simulink model "p_damp_model_p_human"  (R2020b)
settings: Solver=VariableStepAuto  StartTime=0.0  StopTime=200  RelTol=1e-3
values from neighbouring files (symbols this model uses):
  A = [[0 1], ... (first row only)    [p_damp.m]
  A1 = [[0 1], ... (first row only)    [p_damp.m]
  B = [0, ... (first row only)    [p_damp.m]
  B1 = [0, ... (first row only)    [p_damp.m]
  Bl = sqrt(b)*alpha    [p_damp.m]
  Br = Bl*1    [p_damp.m]
  C = [[1 0], ... (first row only)    [p_damp.m]
  C1 = [[1 0], ... (first row only)    [p_damp.m]
  D = [0, ... (first row only)    [p_damp.m]
  D1 = [0, ... (first row only)    [p_damp.m]
  Kl = 0.4    [p_damp.m]
  Kr = 1.1*Kl    (= 0.44)    [p_damp.m]
  stp = 10    [p_damp.m]
  stp_end = 25    [p_damp.m]
  stp_start = 5    [p_damp.m]
  Tl = 2.5    [p_damp.m]
  torque_ratio = 5/8    (= 0.625)    [p_damp.m]
  Tr = 2.5    [p_damp.m]
settings Model: Creator=tammer  LastModifiedBy=tammer

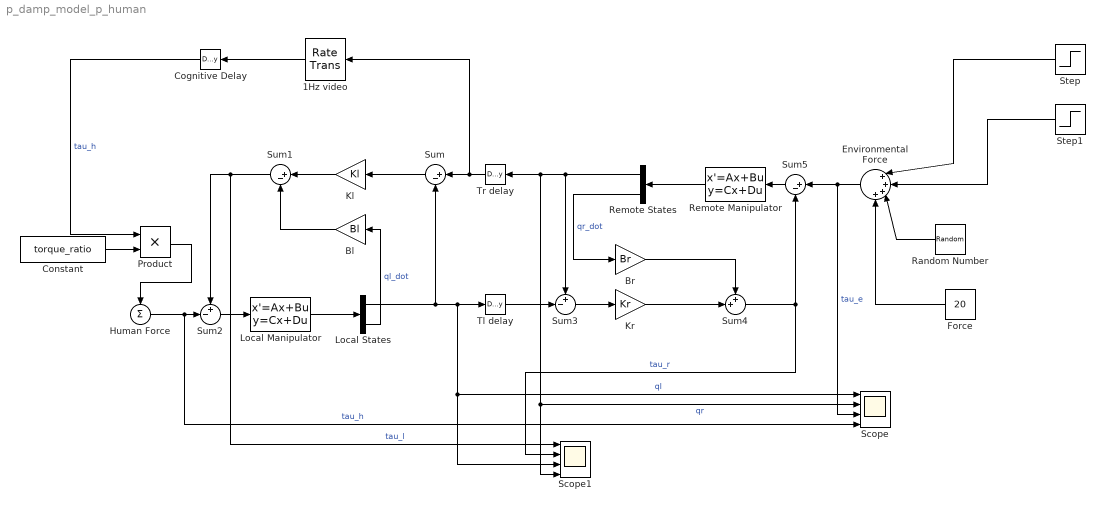
== system p_damp_model_p_human ==
  1Hz video : RateTransition  OutPortSampleTime=1
  Bl : Gain  Gain=Bl
  Br : Gain  Gain=Br
  Cognitive Delay : TransportDelay  DelayTime=.5
  Constant : Constant  Value=torque_ratio
  Environmental Force : Sum  Inputs=|++++
  Force : Constant  Value=20
  Human Force : Sum  Inputs=+|
  Kl : Gain  Gain=Kl
  Kr : Gain  Gain=Kr
  Local Manipulator : StateSpace  A=A  B=B  C=C  D=D  InitialCondition=0
  Local States : Demux  Outputs=2
  Product : Product
  Random Number : RandomNumber  Variance=2  Seed=6  SampleTime=0.1
  Remote Manipulator : StateSpace  A=A1  B=B1  C=C1  D=D1  InitialCondition=0
  Remote States : Demux  Outputs=2
  Scope : Scope  NumInputPorts=4
  Scope1 : Scope  NumInputPorts=4
  Step : Step  Time=stp_start  After=stp  SampleTime=0
  Step1 : Step  Time=stp_end  After=-stp  SampleTime=0
  Sum : Sum  Inputs=|+-
  Sum1 : Sum  Inputs=|+-
  Sum2 : Sum  Inputs=+-|
  Sum3 : Sum  Inputs=+-|
  Sum4 : Sum  Inputs=++|
  Sum5 : Sum  Inputs=|+-
  Tl delay : TransportDelay  DelayTime=Tl
  Tr delay : TransportDelay  DelayTime=Tr
  wires:
  Kl/1 -> Sum1/1
  Sum/1 -> Kl/1
  Sum3/1 -> Kr/1
  Environmental Force/1 -> Scope/3, Sum5/1  "tau_e"
  Tl delay/1 -> Sum3/2
  Sum2/1 -> Local Manipulator/1
  Sum5/1 -> Remote Manipulator/1
  Remote Manipulator/1 -> Remote States/1
  Remote States/1 -> Scope1/4, Scope/2, Tr delay/1, Sum3/1  "qr"
  Local Manipulator/1 -> Local States/1
  Local States/1 -> Tl delay/1, Scope1/3, Scope/1, Sum/2  "ql"
  Bl/1 -> Sum1/2
  Sum1/1 -> Sum2/1, Scope1/1  "tau_l"
  Kr/1 -> Sum4/2
  Br/1 -> Sum4/1
  Sum4/1 -> Sum5/2, Scope1/2  "tau_r"
  Local States/2 -> Bl/1  "ql_dot"
  Remote States/2 -> Br/1  "qr_dot"
  Human Force/1 -> Scope/4, Sum2/2  "tau_h"
  Random Number/1 -> Environmental Force/3
  Step/1 -> Environmental Force/1
  Product/1 -> Human Force/1
  Constant/1 -> Product/2
  Tr delay/1 -> 1Hz video/1, Sum/1
  Step1/1 -> Environmental Force/2
  Force/1 -> Environmental Force/4
  1Hz video/1 -> Cognitive Delay/1
  Cognitive Delay/1 -> Product/1  "tau_h"
